simulink model "e05"  (R2023b)
settings: Solver=FixedStepAuto  StartTime=0.0  StopTime=20  FixedStep=1e-4  RelTol=1e-3
values from neighbouring files (symbols this model uses):
  Ad1 = s1.A    [e01.m]
  Ad2 = s2.A    [e01.m]
  Ad3 = s3.A    [e01.m]
  Bd1 = s1.B    [e01.m]
  Bd2 = s2.B    [e01.m]
  Bd3 = s3.B    [e01.m]
  C1 = 1e-3    (= 0.001)    [e01.m]
  Cd1 = s1.C    [e01.m]
  Cd2 = s2.C    [e01.m]
  Cd3 = s3.C    [e01.m]
  Dd1 = s1.D    [e01.m]
  Dd2 = s2.D    [e01.m]
  Dd3 = s3.D    [e01.m]
  Ld1 = (place(Ad1',Cd1',p))'    [e01.m]
  Ld2 = (place(Ad2',Cd2',p))'    [e01.m]
  Ld3 = (place(Ad3',Cd3',p))'    [e01.m]
  R1 = 1e3    (= 1000)    [e01.m]
  R2 = 2e3    (= 2000)    [e01.m]
  Ts = 1/fs    (= 0.001)    [e01.m]
libraries: fl_lib x27, nesl_utility x15, ee_lib x3, simulink x3
settings Model: Creator=jitbi  LastModifiedBy=Anirvan Krishna

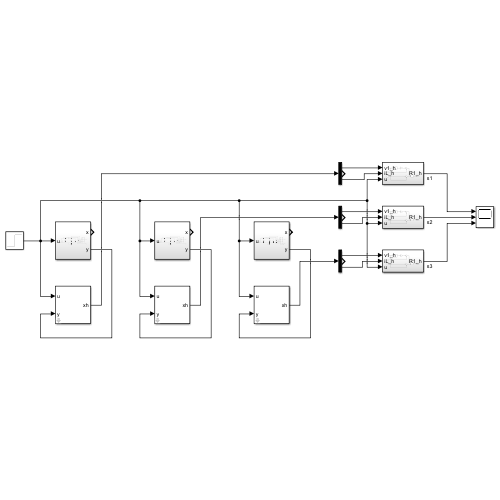
[thumbnail: Simulink's stored preview of the top-level diagram]
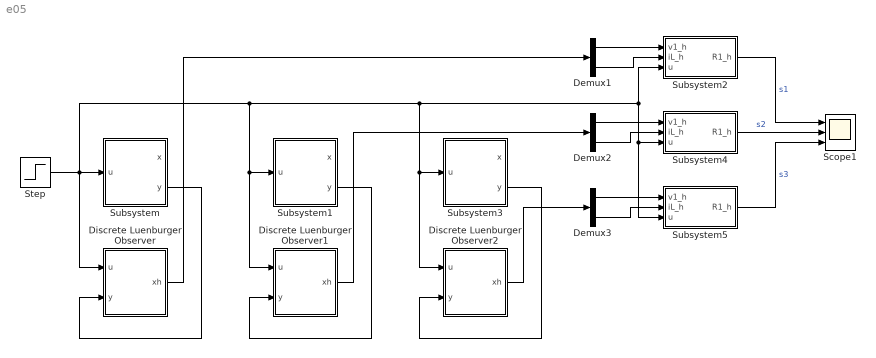
== system e05 ==
  Demux1 : Demux  Outputs=3
  Demux2 : Demux  Outputs=3
  Demux3 : Demux  Outputs=3
  Discrete Luenburger Observer : Subsystem  mask{Ad0=Ad1, Bd0=Bd1, Cd0=Cd1, Dd0=Dd1, Ld0=Ld1}
      mask prompts: Ad0 "Ad"; Bd0 "Bd"; Cd0 "Cd"; Dd0 "Dd"; Ld0 "Ld"
  Discrete Luenburger Observer1 : Subsystem  mask{Ad0=Ad2, Bd0=Bd2, Cd0=Cd2, Dd0=Dd2, Ld0=Ld2}
      mask prompts: Ad0 "Ad"; Bd0 "Bd"; Cd0 "Cd"; Dd0 "Dd"; Ld0 "Ld"
  Discrete Luenburger Observer2 : Subsystem  mask{Ad0=Ad3, Bd0=Bd3, Cd0=Cd3, Dd0=Dd3, Ld0=Ld3}
      mask prompts: Ad0 "Ad"; Bd0 "Bd"; Cd0 "Cd"; Dd0 "Dd"; Ld0 "Ld"
  Scope1 : Scope  NumInputPorts=3
  Step : Step  SampleTime=0
  Subsystem : Subsystem
  Subsystem1 : Subsystem
  Subsystem2 : Subsystem
  Subsystem3 : Subsystem
  Subsystem4 : Subsystem
  Subsystem5 : Subsystem
  wires:
  Subsystem/2(y) -> Discrete Luenburger Observer/2(y)
  Demux1/1 -> Subsystem2/1(v1_h)
  Demux1/3 -> Subsystem2/2(iL_h)
  Subsystem2/1(R1_h) -> Scope1/1  "s1"
  Subsystem1/2(y) -> Discrete Luenburger Observer1/2(y)
  Subsystem3/2(y) -> Discrete Luenburger Observer2/2(y)
  Step/1 -> Discrete Luenburger Observer/1(u), Subsystem2/3(u), Subsystem4/3(u), Subsystem5/3(u), Subsystem3/1(u), Discrete Luenburger Observer2/1(u), Discrete Luenburger Observer1/1(u), Subsystem1/1(u), Subsystem/1(u)
  Demux2/1 -> Subsystem4/1(v1_h)
  Demux2/3 -> Subsystem4/2(iL_h)
  Demux3/1 -> Subsystem5/1(v1_h)
  Demux3/3 -> Subsystem5/2(iL_h)
  Discrete Luenburger Observer/1(xh) -> Demux1/1
  Discrete Luenburger Observer1/1(xh) -> Demux2/1
  Discrete Luenburger Observer2/1(xh) -> Demux3/1
  Subsystem4/1(R1_h) -> Scope1/2  "s2"
  Subsystem5/1(R1_h) -> Scope1/3  "s3"

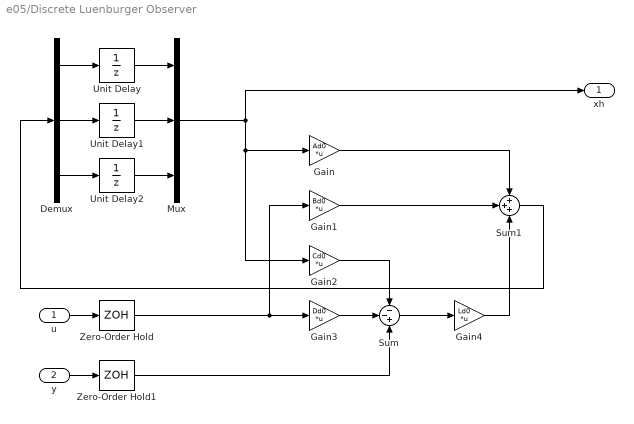
== system e05/Discrete Luenburger Observer ==
  u : Inport
  y : Inport  Port=2
  Demux : Demux  Outputs=3
  Gain : Gain  Gain=Ad0  Multiplication=Matrix(K*u)
  Gain1 : Gain  Gain=Bd0  Multiplication=Matrix(K*u)
  Gain2 : Gain  Gain=Cd0  Multiplication=Matrix(K*u)
  Gain3 : Gain  Gain=Dd0  Multiplication=Matrix(K*u)
  Gain4 : Gain  Gain=Ld0  Multiplication=Matrix(K*u)
  Mux : Mux  Inputs=3
  Sum : Sum  Inputs=--+
  Sum1 : Sum  Inputs=+++
  Unit Delay : UnitDelay  SampleTime=Ts  HasFrameUpgradeWarning=on
  Unit Delay1 : UnitDelay  SampleTime=Ts  HasFrameUpgradeWarning=on
  Unit Delay2 : UnitDelay  SampleTime=Ts  HasFrameUpgradeWarning=on
  Zero-Order Hold : ZeroOrderHold  SampleTime=Ts
  Zero-Order Hold1 : ZeroOrderHold  SampleTime=Ts
  xh : Outport
  wires:
  y/1 -> Zero-Order Hold1/1
  Gain3/1 -> Sum/2
  Unit Delay1/1 -> Mux/2
  Unit Delay/1 -> Mux/1
  Unit Delay2/1 -> Mux/3
  u/1 -> Zero-Order Hold/1
  Gain4/1 -> Sum1/3
  Demux/2 -> Unit Delay1/1
  Zero-Order Hold/1 -> Gain3/1, Gain1/1
  Mux/1 -> Gain2/1, Gain/1, xh/1
  Demux/3 -> Unit Delay2/1
  Gain/1 -> Sum1/1
  Demux/1 -> Unit Delay/1
  Zero-Order Hold1/1 -> Sum/3
  Gain1/1 -> Sum1/2
  Sum/1 -> Gain4/1
  Gain2/1 -> Sum/1
  Sum1/1 -> Demux/1

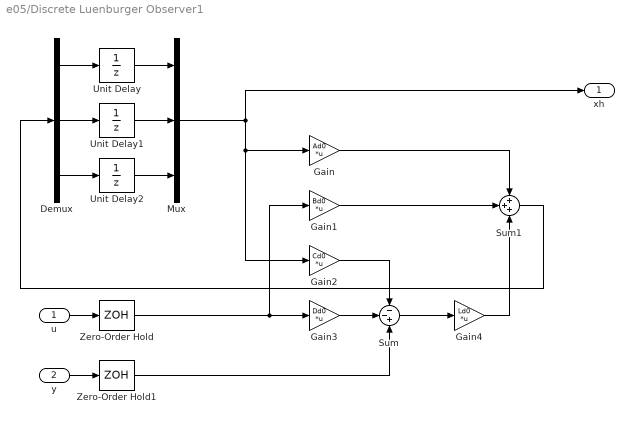
== system e05/Discrete Luenburger Observer1 ==
  u : Inport
  y : Inport  Port=2
  Demux : Demux  Outputs=3
  Gain : Gain  Gain=Ad0  Multiplication=Matrix(K*u)
  Gain1 : Gain  Gain=Bd0  Multiplication=Matrix(K*u)
  Gain2 : Gain  Gain=Cd0  Multiplication=Matrix(K*u)
  Gain3 : Gain  Gain=Dd0  Multiplication=Matrix(K*u)
  Gain4 : Gain  Gain=Ld0  Multiplication=Matrix(K*u)
  Mux : Mux  Inputs=3
  Sum : Sum  Inputs=--+
  Sum1 : Sum  Inputs=+++
  Unit Delay : UnitDelay  SampleTime=Ts  HasFrameUpgradeWarning=on
  Unit Delay1 : UnitDelay  SampleTime=Ts  HasFrameUpgradeWarning=on
  Unit Delay2 : UnitDelay  SampleTime=Ts  HasFrameUpgradeWarning=on
  Zero-Order Hold : ZeroOrderHold  SampleTime=Ts
  Zero-Order Hold1 : ZeroOrderHold  SampleTime=Ts
  xh : Outport
  wires:
  Sum1/1 -> Demux/1
  Gain2/1 -> Sum/1
  Sum/1 -> Gain4/1
  Gain1/1 -> Sum1/2
  Zero-Order Hold1/1 -> Sum/3
  Demux/1 -> Unit Delay/1
  Gain/1 -> Sum1/1
  Demux/3 -> Unit Delay2/1
  Mux/1 -> xh/1, Gain/1, Gain2/1
  Zero-Order Hold/1 -> Gain1/1, Gain3/1
  Demux/2 -> Unit Delay1/1
  Gain4/1 -> Sum1/3
  u/1 -> Zero-Order Hold/1
  Unit Delay2/1 -> Mux/3
  Unit Delay/1 -> Mux/1
  Unit Delay1/1 -> Mux/2
  Gain3/1 -> Sum/2
  y/1 -> Zero-Order Hold1/1

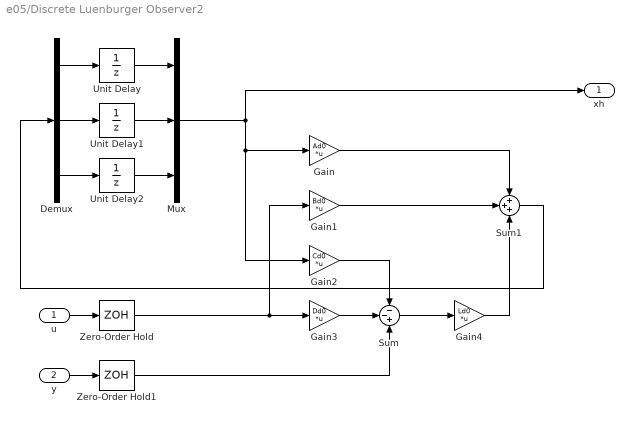
== system e05/Discrete Luenburger Observer2 ==
  u : Inport
  y : Inport  Port=2
  Demux : Demux  Outputs=3
  Gain : Gain  Gain=Ad0  Multiplication=Matrix(K*u)
  Gain1 : Gain  Gain=Bd0  Multiplication=Matrix(K*u)
  Gain2 : Gain  Gain=Cd0  Multiplication=Matrix(K*u)
  Gain3 : Gain  Gain=Dd0  Multiplication=Matrix(K*u)
  Gain4 : Gain  Gain=Ld0  Multiplication=Matrix(K*u)
  Mux : Mux  Inputs=3
  Sum : Sum  Inputs=--+
  Sum1 : Sum  Inputs=+++
  Unit Delay : UnitDelay  SampleTime=Ts  HasFrameUpgradeWarning=on
  Unit Delay1 : UnitDelay  SampleTime=Ts  HasFrameUpgradeWarning=on
  Unit Delay2 : UnitDelay  SampleTime=Ts  HasFrameUpgradeWarning=on
  Zero-Order Hold : ZeroOrderHold  SampleTime=Ts
  Zero-Order Hold1 : ZeroOrderHold  SampleTime=Ts
  xh : Outport
  wires:
  y/1 -> Zero-Order Hold1/1
  Gain3/1 -> Sum/2
  Unit Delay1/1 -> Mux/2
  Unit Delay/1 -> Mux/1
  Unit Delay2/1 -> Mux/3
  u/1 -> Zero-Order Hold/1
  Gain4/1 -> Sum1/3
  Demux/2 -> Unit Delay1/1
  Zero-Order Hold/1 -> Gain3/1, Gain1/1
  Mux/1 -> Gain2/1, Gain/1, xh/1
  Demux/3 -> Unit Delay2/1
  Gain/1 -> Sum1/1
  Demux/1 -> Unit Delay/1
  Zero-Order Hold1/1 -> Sum/3
  Gain1/1 -> Sum1/2
  Sum/1 -> Gain4/1
  Gain2/1 -> Sum/1
  Sum1/1 -> Demux/1

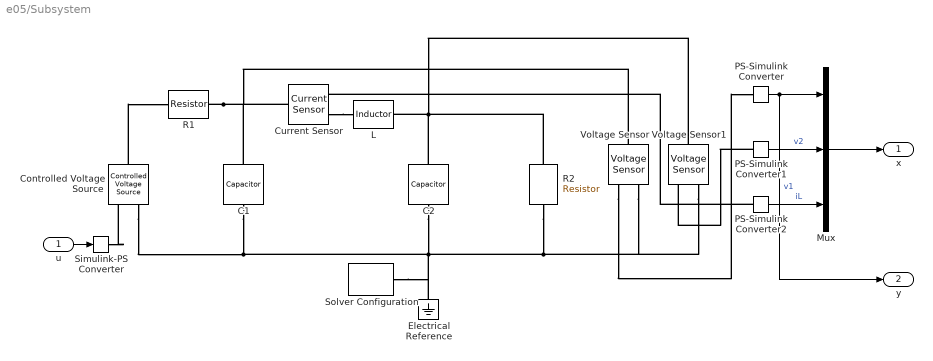
== system e05/Subsystem ==
  u : Inport
  C1 : fl_lib/Electrical/Electrical Elements/Capacitor  c=C1 F  r=1e-6 Ohm  g=0 1/Ohm  i_specify=off  i_priority=None  i=0 A  i_nominal_specify=off  i_nominal_unit=A  i_nominal_value=1  v_specify=off  v_priority=None  v=0 V  v_nominal_specify=off  v_nominal_unit=V  v_nominal_value=1  vc_specify=off  vc_priority=High  vc=0 V  vc_nominal_specify=off  vc_nominal_unit=V  vc_nominal_value=1
  C2 : fl_lib/Electrical/Electrical Elements/Capacitor  c=C2 F  r=1e-6 Ohm  g=0 1/Ohm  i_specify=off  i_priority=None  i=0 A  i_nominal_specify=off  i_nominal_unit=A  i_nominal_value=1  v_specify=off  v_priority=None  v=0 V  v_nominal_specify=off  v_nominal_unit=V  v_nominal_value=1  vc_specify=off  vc_priority=High  vc=0 V  vc_nominal_specify=off  vc_nominal_unit=V  vc_nominal_value=1
  Controlled Voltage Source : fl_lib/Electrical/Electrical Sources/Controlled Voltage Source
  Current Sensor : fl_lib/Electrical/Electrical Sensors/Current Sensor
  Electrical Reference : fl_lib/Electrical/Electrical Elements/Electrical Reference
  L : ee_lib/Passive/Inductor  l=L H  enable_L_tol=ee.enum.toleranceApplication.none  L_tol=20  tol_distribution=ee.enum.toleranceDistribution.uniform  nSigma=4  r=0 Ohm  g=1e-9 1/Ohm  enable_operating_limits=ee.enum.enable.no  operating_limit_action=ee.enum.passive.reportOpLim.warn  max_working_current=1 A  power_rating=1 W  enable_faults=ee.enum.enable.no  fault_action=simscape.enum.assert.action.none  lambdaPercent=50  k_faulted=0.9999  turnsShort=ee.enum.passive.inductor.turnsShortOption.no  openCct=ee.enum.enable.no  groundShort=ee.enum.passive.inductor.groundShortOption.no  groundShortG=0 1/Ohm  tau_fault=1e-3 s  fault_trigger=ee.enum.faults.faultTrigger.temporal  t_fault=1 s  max_permissible_voltage=100 V  n_fail_on_voltage=1  max_permissible_current=1 A  t_fail_on_current=1 s  i_L_specify=off  i_L_priority=High  i_L=0 A  i_L_nominal_specify=off  i_L_nominal_unit=A  i_L_nominal_value=1
  Mux : Mux  Inputs=3
  PS-Simulink Converter : nesl_utility/PS-Simulink Converter  PhysicalDomain=network_engine_domain  SubClassName=ps_output  LeftPortType=input  RightPortType=output  PseudoPeriodic=off  Frequencies=[]  VectorFormat=inherit  Unit=inherit  AffineConversion=off
  PS-Simulink Converter1 : nesl_utility/PS-Simulink Converter  PhysicalDomain=network_engine_domain  SubClassName=ps_output  LeftPortType=input  RightPortType=output  PseudoPeriodic=off  Frequencies=[]  VectorFormat=inherit  Unit=inherit  AffineConversion=off
  PS-Simulink Converter2 : nesl_utility/PS-Simulink Converter  PhysicalDomain=network_engine_domain  SubClassName=ps_output  LeftPortType=input  RightPortType=output  PseudoPeriodic=off  Frequencies=[]  VectorFormat=inherit  Unit=inherit  AffineConversion=off
  R1 : fl_lib/Electrical/Electrical Elements/Resistor  R=R1 Ohm  i_specify=off  i_priority=None  i=0 A  i_nominal_specify=off  i_nominal_unit=A  i_nominal_value=1  v_specify=off  v_priority=None  v=0 V  v_nominal_specify=off  v_nominal_unit=V  v_nominal_value=1
  R2 : fl_lib/Electrical/Electrical Elements/Resistor  R=R2 Ohm  i_specify=off  i_priority=None  i=0 A  i_nominal_specify=off  i_nominal_unit=A  i_nominal_value=1  v_specify=off  v_priority=None  v=0 V  v_nominal_specify=off  v_nominal_unit=V  v_nominal_value=1
  Simulink-PS Converter : nesl_utility/Simulink-PS Converter  PhysicalDomain=network_engine_domain  SubClassName=ps_input  LeftPortType=input  RightPortType=output  PseudoPeriodic=off  Frequencies=[]  NoiseDistribution=none  NoiseParameters=[]  Unit=1  AffineConversion=off  FilteringAndDerivatives=provide  SimscapeFilterOrder=1  InputFilterTimeConstant=0.001  UdotUserProvided=0
  Solver Configuration : nesl_utility/Solver Configuration  PhysicalDomain=network_engine_domain  SubClassName=solver  LeftPortType=input  RightPortType=generic  Tones=[]  Harmonics=[]  SimulateNoise=off  Profile=off  UseLocalSampling=off  EnableSwitchedLinearOptims=on  FrequencyDomain=off  UseCCode=off  RelTol=0.001  AbsTol=0.001  MinStep=1e-09  ToWorkspace=off  RevertToSquareIcSolve=off  NumHomotopyIterations=100  PhasorMode=off  PhasorModeNumHarmonics=1  ConsistencySolver=NEWTON_XTOL_AFTER_FTOL  IndexReductionMethod=DerivativeReplacement  DoDC=off  ResidualTolerance=1e-09  ConsistencyTolSource=GLOBAL  ConsistencyAbsTol=0.001  ConsistencyRelTol=0.001  ConsistencyTolFactor=0.001  UseLocalSolver=off  LocalSolverChoice=NE_BACKWARD_EULER_ADVANCER  ResolveIndetEquations=on  FunctionEvalNumThread=1  LocalSolverSampleTime=0.001  DoFixedCost=off  MaxNonlinIter=3  MaxModeIter=2  ComputeImpulses=off  ImpulseIterations=2  LinearAlgebra=auto  LinearAlgebraNumThread=0  EquationFormulation=NE_TIME_EF  DelaysMemoryBudget=1024  AutomaticFiltering=on  FilteringTimeConstant=0.001  PartitionStorageMethod=AS_NEEDED  PartitionMemoryBudget=1024  PartitionMethod=ROBUST  MultibodyUseLocalSolver=off  MultibodyLocalSolverChoice=ODE1  MultibodyLocalSolverSampleTime=0.001
  Voltage Sensor : fl_lib/Electrical/Electrical Sensors/Voltage Sensor
  Voltage Sensor1 : fl_lib/Electrical/Electrical Sensors/Voltage Sensor
  x : Outport
  y : Outport  Port=2
  wires:
  PS-Simulink Converter1/1 -> Mux/2  "v2"
  u/1 -> Simulink-PS Converter/1
  PS-Simulink Converter/1 -> y/1, Mux/1  "v1"
  PS-Simulink Converter2/1 -> Mux/3  "iL"
  Mux/1 -> x/1
  connections:
  Controlled Voltage Source/RConn2 -- Solver Configuration/RConn1 -- Electrical Reference/LConn1 -- R2/RConn1 -- Voltage Sensor1/RConn2 -- Voltage Sensor/RConn2 -- C2/RConn1 -- C1/RConn1
  Simulink-PS Converter/RConn1 -- Controlled Voltage Source/RConn1
  C2/LConn1 -- R2/LConn1 -- Voltage Sensor1/LConn1 -- L/RConn1
  Controlled Voltage Source/LConn1 -- R1/LConn1
  R1/RConn1 -- C1/LConn1 -- Current Sensor/LConn1 -- Voltage Sensor/LConn1
  PS-Simulink Converter1/LConn1 -- Voltage Sensor1/RConn1
  PS-Simulink Converter2/LConn1 -- Current Sensor/RConn1
  Current Sensor/RConn2 -- L/LConn1
  Voltage Sensor/RConn1 -- PS-Simulink Converter/LConn1

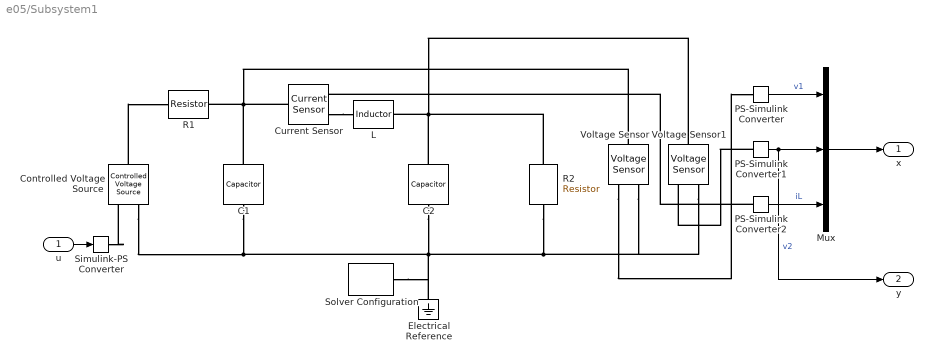
== system e05/Subsystem1 ==
  u : Inport
  C1 : fl_lib/Electrical/Electrical Elements/Capacitor  c=C1 F  r=1e-6 Ohm  g=0 1/Ohm  i_specify=off  i_priority=None  i=0 A  i_nominal_specify=off  i_nominal_unit=A  i_nominal_value=1  v_specify=off  v_priority=None  v=0 V  v_nominal_specify=off  v_nominal_unit=V  v_nominal_value=1  vc_specify=off  vc_priority=High  vc=0 V  vc_nominal_specify=off  vc_nominal_unit=V  vc_nominal_value=1
  C2 : fl_lib/Electrical/Electrical Elements/Capacitor  c=C2 F  r=1e-6 Ohm  g=0 1/Ohm  i_specify=off  i_priority=None  i=0 A  i_nominal_specify=off  i_nominal_unit=A  i_nominal_value=1  v_specify=off  v_priority=None  v=0 V  v_nominal_specify=off  v_nominal_unit=V  v_nominal_value=1  vc_specify=off  vc_priority=High  vc=0 V  vc_nominal_specify=off  vc_nominal_unit=V  vc_nominal_value=1
  Controlled Voltage Source : fl_lib/Electrical/Electrical Sources/Controlled Voltage Source
  Current Sensor : fl_lib/Electrical/Electrical Sensors/Current Sensor
  Electrical Reference : fl_lib/Electrical/Electrical Elements/Electrical Reference
  L : ee_lib/Passive/Inductor  l=L H  enable_L_tol=ee.enum.toleranceApplication.none  L_tol=20  tol_distribution=ee.enum.toleranceDistribution.uniform  nSigma=4  r=0 Ohm  g=1e-9 1/Ohm  enable_operating_limits=ee.enum.enable.no  operating_limit_action=ee.enum.passive.reportOpLim.warn  max_working_current=1 A  power_rating=1 W  enable_faults=ee.enum.enable.no  fault_action=simscape.enum.assert.action.none  lambdaPercent=50  k_faulted=0.9999  turnsShort=ee.enum.passive.inductor.turnsShortOption.no  openCct=ee.enum.enable.no  groundShort=ee.enum.passive.inductor.groundShortOption.no  groundShortG=0 1/Ohm  tau_fault=1e-3 s  fault_trigger=ee.enum.faults.faultTrigger.temporal  t_fault=1 s  max_permissible_voltage=100 V  n_fail_on_voltage=1  max_permissible_current=1 A  t_fail_on_current=1 s  i_L_specify=off  i_L_priority=High  i_L=0 A  i_L_nominal_specify=off  i_L_nominal_unit=A  i_L_nominal_value=1
  Mux : Mux  Inputs=3
  PS-Simulink Converter : nesl_utility/PS-Simulink Converter  PhysicalDomain=network_engine_domain  SubClassName=ps_output  LeftPortType=input  RightPortType=output  PseudoPeriodic=off  Frequencies=[]  VectorFormat=inherit  Unit=inherit  AffineConversion=off
  PS-Simulink Converter1 : nesl_utility/PS-Simulink Converter  PhysicalDomain=network_engine_domain  SubClassName=ps_output  LeftPortType=input  RightPortType=output  PseudoPeriodic=off  Frequencies=[]  VectorFormat=inherit  Unit=inherit  AffineConversion=off
  PS-Simulink Converter2 : nesl_utility/PS-Simulink Converter  PhysicalDomain=network_engine_domain  SubClassName=ps_output  LeftPortType=input  RightPortType=output  PseudoPeriodic=off  Frequencies=[]  VectorFormat=inherit  Unit=inherit  AffineConversion=off
  R1 : fl_lib/Electrical/Electrical Elements/Resistor  R=R1 Ohm  i_specify=off  i_priority=None  i=0 A  i_nominal_specify=off  i_nominal_unit=A  i_nominal_value=1  v_specify=off  v_priority=None  v=0 V  v_nominal_specify=off  v_nominal_unit=V  v_nominal_value=1
  R2 : fl_lib/Electrical/Electrical Elements/Resistor  R=R2 Ohm  i_specify=off  i_priority=None  i=0 A  i_nominal_specify=off  i_nominal_unit=A  i_nominal_value=1  v_specify=off  v_priority=None  v=0 V  v_nominal_specify=off  v_nominal_unit=V  v_nominal_value=1
  Simulink-PS Converter : nesl_utility/Simulink-PS Converter  PhysicalDomain=network_engine_domain  SubClassName=ps_input  LeftPortType=input  RightPortType=output  PseudoPeriodic=off  Frequencies=[]  NoiseDistribution=none  NoiseParameters=[]  Unit=1  AffineConversion=off  FilteringAndDerivatives=provide  SimscapeFilterOrder=1  InputFilterTimeConstant=0.001  UdotUserProvided=0
  Solver Configuration : nesl_utility/Solver Configuration  PhysicalDomain=network_engine_domain  SubClassName=solver  LeftPortType=input  RightPortType=generic  Tones=[]  Harmonics=[]  SimulateNoise=off  Profile=off  UseLocalSampling=off  EnableSwitchedLinearOptims=on  FrequencyDomain=off  UseCCode=off  RelTol=0.001  AbsTol=0.001  MinStep=1e-09  ToWorkspace=off  RevertToSquareIcSolve=off  NumHomotopyIterations=100  PhasorMode=off  PhasorModeNumHarmonics=1  ConsistencySolver=NEWTON_XTOL_AFTER_FTOL  IndexReductionMethod=DerivativeReplacement  DoDC=off  ResidualTolerance=1e-09  ConsistencyTolSource=GLOBAL  ConsistencyAbsTol=0.001  ConsistencyRelTol=0.001  ConsistencyTolFactor=0.001  UseLocalSolver=off  LocalSolverChoice=NE_BACKWARD_EULER_ADVANCER  ResolveIndetEquations=on  FunctionEvalNumThread=1  LocalSolverSampleTime=0.001  DoFixedCost=off  MaxNonlinIter=3  MaxModeIter=2  ComputeImpulses=off  ImpulseIterations=2  LinearAlgebra=auto  LinearAlgebraNumThread=0  EquationFormulation=NE_TIME_EF  DelaysMemoryBudget=1024  AutomaticFiltering=on  FilteringTimeConstant=0.001  PartitionStorageMethod=AS_NEEDED  PartitionMemoryBudget=1024  PartitionMethod=ROBUST  MultibodyUseLocalSolver=off  MultibodyLocalSolverChoice=ODE1  MultibodyLocalSolverSampleTime=0.001
  Voltage Sensor : fl_lib/Electrical/Electrical Sensors/Voltage Sensor
  Voltage Sensor1 : fl_lib/Electrical/Electrical Sensors/Voltage Sensor
  x : Outport
  y : Outport  Port=2
  wires:
  Mux/1 -> x/1
  PS-Simulink Converter2/1 -> Mux/3  "iL"
  PS-Simulink Converter/1 -> Mux/1  "v1"
  u/1 -> Simulink-PS Converter/1
  PS-Simulink Converter1/1 -> Mux/2, y/1  "v2"
  connections:
  Voltage Sensor/RConn1 -- PS-Simulink Converter/LConn1
  Current Sensor/RConn2 -- L/LConn1
  PS-Simulink Converter2/LConn1 -- Current Sensor/RConn1
  PS-Simulink Converter1/LConn1 -- Voltage Sensor1/RConn1
  Voltage Sensor/LConn1 -- Current Sensor/LConn1 -- C1/LConn1 -- R1/RConn1
  Controlled Voltage Source/LConn1 -- R1/LConn1
  R2/LConn1 -- L/RConn1 -- Voltage Sensor1/LConn1 -- C2/LConn1
  Simulink-PS Converter/RConn1 -- Controlled Voltage Source/RConn1
  R2/RConn1 -- Voltage Sensor/RConn2 -- Voltage Sensor1/RConn2 -- C2/RConn1 -- Electrical Reference/LConn1 -- Solver Configuration/RConn1 -- C1/RConn1 -- Controlled Voltage Source/RConn2

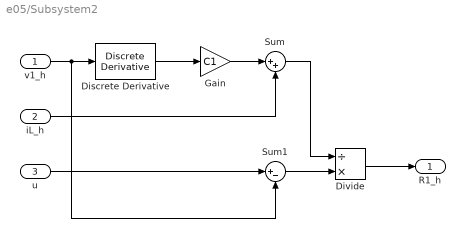
== system e05/Subsystem2 ==
  v1_h : Inport
  iL_h : Inport  Port=2
  u : Inport  Port=3
  Discrete Derivative : simulink/Discrete/Discrete Derivative  gainval=1.0  ICPrevScaledInput=0.0  OutMin=[]  OutMax=[]  OutDataType=fixdt(1, 16)  OutScaling=2^-10  DoSatur=off
  Divide : Product  Inputs=/*
  Gain : Gain  Gain=C1
  Sum : Sum  Inputs=|++
  Sum1 : Sum  Inputs=|+-
  R1_h : Outport
  wires:
  v1_h/1 -> Discrete Derivative/1, Sum1/2
  Discrete Derivative/1 -> Gain/1
  Gain/1 -> Sum/1
  iL_h/1 -> Sum/2
  u/1 -> Sum1/1
  Sum1/1 -> Divide/2
  Sum/1 -> Divide/1
  Divide/1 -> R1_h/1

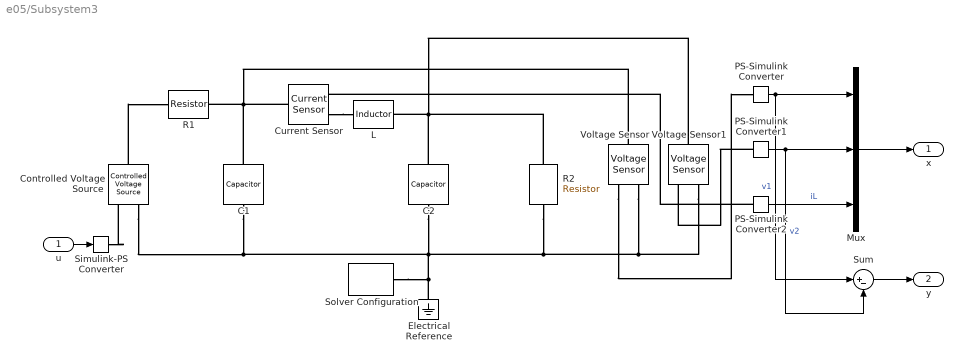
== system e05/Subsystem3 ==
  u : Inport
  C1 : fl_lib/Electrical/Electrical Elements/Capacitor  c=C1 F  r=1e-6 Ohm  g=0 1/Ohm  i_specify=off  i_priority=None  i=0 A  i_nominal_specify=off  i_nominal_unit=A  i_nominal_value=1  v_specify=off  v_priority=None  v=0 V  v_nominal_specify=off  v_nominal_unit=V  v_nominal_value=1  vc_specify=off  vc_priority=High  vc=0 V  vc_nominal_specify=off  vc_nominal_unit=V  vc_nominal_value=1
  C2 : fl_lib/Electrical/Electrical Elements/Capacitor  c=C2 F  r=1e-6 Ohm  g=0 1/Ohm  i_specify=off  i_priority=None  i=0 A  i_nominal_specify=off  i_nominal_unit=A  i_nominal_value=1  v_specify=off  v_priority=None  v=0 V  v_nominal_specify=off  v_nominal_unit=V  v_nominal_value=1  vc_specify=off  vc_priority=High  vc=0 V  vc_nominal_specify=off  vc_nominal_unit=V  vc_nominal_value=1
  Controlled Voltage Source : fl_lib/Electrical/Electrical Sources/Controlled Voltage Source
  Current Sensor : fl_lib/Electrical/Electrical Sensors/Current Sensor
  Electrical Reference : fl_lib/Electrical/Electrical Elements/Electrical Reference
  L : ee_lib/Passive/Inductor  l=L H  enable_L_tol=ee.enum.toleranceApplication.none  L_tol=20  tol_distribution=ee.enum.toleranceDistribution.uniform  nSigma=4  r=0 Ohm  g=1e-9 1/Ohm  enable_operating_limits=ee.enum.enable.no  operating_limit_action=ee.enum.passive.reportOpLim.warn  max_working_current=1 A  power_rating=1 W  enable_faults=ee.enum.enable.no  fault_action=simscape.enum.assert.action.none  lambdaPercent=50  k_faulted=0.9999  turnsShort=ee.enum.passive.inductor.turnsShortOption.no  openCct=ee.enum.enable.no  groundShort=ee.enum.passive.inductor.groundShortOption.no  groundShortG=0 1/Ohm  tau_fault=1e-3 s  fault_trigger=ee.enum.faults.faultTrigger.temporal  t_fault=1 s  max_permissible_voltage=100 V  n_fail_on_voltage=1  max_permissible_current=1 A  t_fail_on_current=1 s  i_L_specify=off  i_L_priority=High  i_L=0 A  i_L_nominal_specify=off  i_L_nominal_unit=A  i_L_nominal_value=1
  Mux : Mux  Inputs=3
  PS-Simulink Converter : nesl_utility/PS-Simulink Converter  PhysicalDomain=network_engine_domain  SubClassName=ps_output  LeftPortType=input  RightPortType=output  PseudoPeriodic=off  Frequencies=[]  VectorFormat=inherit  Unit=inherit  AffineConversion=off
  PS-Simulink Converter1 : nesl_utility/PS-Simulink Converter  PhysicalDomain=network_engine_domain  SubClassName=ps_output  LeftPortType=input  RightPortType=output  PseudoPeriodic=off  Frequencies=[]  VectorFormat=inherit  Unit=inherit  AffineConversion=off
  PS-Simulink Converter2 : nesl_utility/PS-Simulink Converter  PhysicalDomain=network_engine_domain  SubClassName=ps_output  LeftPortType=input  RightPortType=output  PseudoPeriodic=off  Frequencies=[]  VectorFormat=inherit  Unit=inherit  AffineConversion=off
  R1 : fl_lib/Electrical/Electrical Elements/Resistor  R=R1 Ohm  i_specify=off  i_priority=None  i=0 A  i_nominal_specify=off  i_nominal_unit=A  i_nominal_value=1  v_specify=off  v_priority=None  v=0 V  v_nominal_specify=off  v_nominal_unit=V  v_nominal_value=1
  R2 : fl_lib/Electrical/Electrical Elements/Resistor  R=R2 Ohm  i_specify=off  i_priority=None  i=0 A  i_nominal_specify=off  i_nominal_unit=A  i_nominal_value=1  v_specify=off  v_priority=None  v=0 V  v_nominal_specify=off  v_nominal_unit=V  v_nominal_value=1
  Simulink-PS Converter : nesl_utility/Simulink-PS Converter  PhysicalDomain=network_engine_domain  SubClassName=ps_input  LeftPortType=input  RightPortType=output  PseudoPeriodic=off  Frequencies=[]  NoiseDistribution=none  NoiseParameters=[]  Unit=1  AffineConversion=off  FilteringAndDerivatives=provide  SimscapeFilterOrder=1  InputFilterTimeConstant=0.001  UdotUserProvided=0
  Solver Configuration : nesl_utility/Solver Configuration  PhysicalDomain=network_engine_domain  SubClassName=solver  LeftPortType=input  RightPortType=generic  Tones=[]  Harmonics=[]  SimulateNoise=off  Profile=off  UseLocalSampling=off  EnableSwitchedLinearOptims=on  FrequencyDomain=off  UseCCode=off  RelTol=0.001  AbsTol=0.001  MinStep=1e-09  ToWorkspace=off  RevertToSquareIcSolve=off  NumHomotopyIterations=100  PhasorMode=off  PhasorModeNumHarmonics=1  ConsistencySolver=NEWTON_XTOL_AFTER_FTOL  IndexReductionMethod=DerivativeReplacement  DoDC=off  ResidualTolerance=1e-09  ConsistencyTolSource=GLOBAL  ConsistencyAbsTol=0.001  ConsistencyRelTol=0.001  ConsistencyTolFactor=0.001  UseLocalSolver=off  LocalSolverChoice=NE_BACKWARD_EULER_ADVANCER  ResolveIndetEquations=on  FunctionEvalNumThread=1  LocalSolverSampleTime=0.001  DoFixedCost=off  MaxNonlinIter=3  MaxModeIter=2  ComputeImpulses=off  ImpulseIterations=2  LinearAlgebra=auto  LinearAlgebraNumThread=0  EquationFormulation=NE_TIME_EF  DelaysMemoryBudget=1024  AutomaticFiltering=on  FilteringTimeConstant=0.001  PartitionStorageMethod=AS_NEEDED  PartitionMemoryBudget=1024  PartitionMethod=ROBUST  MultibodyUseLocalSolver=off  MultibodyLocalSolverChoice=ODE1  MultibodyLocalSolverSampleTime=0.001
  Sum : Sum  Inputs=|+-
  Voltage Sensor : fl_lib/Electrical/Electrical Sensors/Voltage Sensor
  Voltage Sensor1 : fl_lib/Electrical/Electrical Sensors/Voltage Sensor
  x : Outport
  y : Outport  Port=2
  wires:
  PS-Simulink Converter1/1 -> Mux/2, Sum/2  "v2"
  u/1 -> Simulink-PS Converter/1
  PS-Simulink Converter/1 -> Mux/1, Sum/1  "v1"
  PS-Simulink Converter2/1 -> Mux/3  "iL"
  Mux/1 -> x/1
  Sum/1 -> y/1
  connections:
  Controlled Voltage Source/RConn2 -- C1/RConn1 -- Solver Configuration/RConn1 -- Electrical Reference/LConn1 -- C2/RConn1 -- Voltage Sensor1/RConn2 -- Voltage Sensor/RConn2 -- R2/RConn1
  Simulink-PS Converter/RConn1 -- Controlled Voltage Source/RConn1
  C2/LConn1 -- Voltage Sensor1/LConn1 -- L/RConn1 -- R2/LConn1
  Controlled Voltage Source/LConn1 -- R1/LConn1
  R1/RConn1 -- C1/LConn1 -- Current Sensor/LConn1 -- Voltage Sensor/LConn1
  PS-Simulink Converter1/LConn1 -- Voltage Sensor1/RConn1
  PS-Simulink Converter2/LConn1 -- Current Sensor/RConn1
  Current Sensor/RConn2 -- L/LConn1
  Voltage Sensor/RConn1 -- PS-Simulink Converter/LConn1

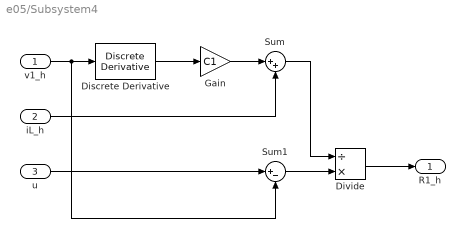
== system e05/Subsystem4 ==
  v1_h : Inport
  iL_h : Inport  Port=2
  u : Inport  Port=3
  Discrete Derivative : simulink/Discrete/Discrete Derivative  gainval=1.0  ICPrevScaledInput=0.0  OutMin=[]  OutMax=[]  OutDataType=fixdt(1, 16)  OutScaling=2^-10  DoSatur=off
  Divide : Product  Inputs=/*
  Gain : Gain  Gain=C1
  Sum : Sum  Inputs=|++
  Sum1 : Sum  Inputs=|+-
  R1_h : Outport
  wires:
  Divide/1 -> R1_h/1
  Sum/1 -> Divide/1
  Sum1/1 -> Divide/2
  u/1 -> Sum1/1
  iL_h/1 -> Sum/2
  Gain/1 -> Sum/1
  Discrete Derivative/1 -> Gain/1
  v1_h/1 -> Sum1/2, Discrete Derivative/1

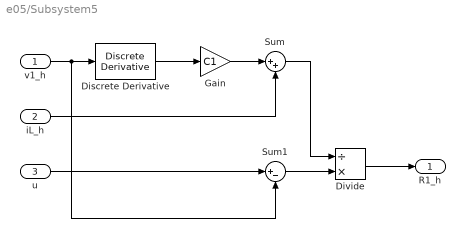
== system e05/Subsystem5 ==
  v1_h : Inport
  iL_h : Inport  Port=2
  u : Inport  Port=3
  Discrete Derivative : simulink/Discrete/Discrete Derivative  gainval=1.0  ICPrevScaledInput=0.0  OutMin=[]  OutMax=[]  OutDataType=fixdt(1, 16)  OutScaling=2^-10  DoSatur=off
  Divide : Product  Inputs=/*
  Gain : Gain  Gain=C1
  Sum : Sum  Inputs=|++
  Sum1 : Sum  Inputs=|+-
  R1_h : Outport
  wires:
  v1_h/1 -> Discrete Derivative/1, Sum1/2
  Discrete Derivative/1 -> Gain/1
  Gain/1 -> Sum/1
  iL_h/1 -> Sum/2
  u/1 -> Sum1/1
  Sum1/1 -> Divide/2
  Sum/1 -> Divide/1
  Divide/1 -> R1_h/1
